simulink model "pre4"  (R2021a)
settings: Solver=VariableStepAuto  StartTime=0.0  StopTime=10.0  RelTol=1e-3
libraries: dsparch4 x3, commsynccomp2 x1, spspowerguiLib x1
settings Model: Creator=Dell  LastModifiedBy=Dell

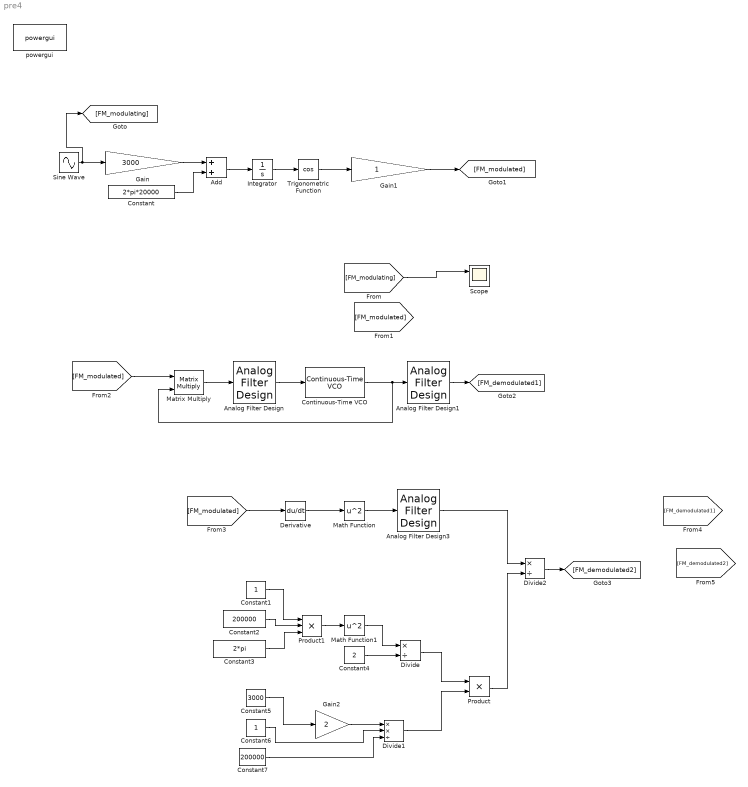
== system pre4 ==
  Add : Sum
  Analog Filter Design : dsparch4/Analog Filter Design  method=Butterworth  filttype=Lowpass  N=8  Wlo=30  Whi=80  Rp=2  Rs=40
  Analog Filter Design1 : dsparch4/Analog Filter Design  method=Butterworth  filttype=Lowpass  N=8  Wlo=30  Whi=80  Rp=2  Rs=40
  Analog Filter Design3 : dsparch4/Analog Filter Design  method=Butterworth  filttype=Bandpass  N=8  Wlo=30  Whi=80  Rp=2  Rs=40
  Constant : Constant  Value=2*pi*20000
  Constant1 : Constant
  Constant2 : Constant  Value=200000
  Constant3 : Constant  Value=2*pi
  Constant4 : Constant  Value=2
  Constant5 : Constant  Value=3000
  Constant6 : Constant
  Constant7 : Constant  Value=200000
  Continuous-Time VCO : commsynccomp2/Continuous-Time VCO  Ac=1  Fc=10  Kc=1  Ph=0
      settings: SourceProductBaseCode=CM
  Derivative : Derivative
  Divide : Product  Inputs=*/
  Divide1 : Product  Inputs=**/
  Divide2 : Product  Inputs=*/
  Gain : Gain  Gain=3000
  Gain1 : Gain
  Gain2 : Gain  Gain=2
  Integrator : Integrator
  Math Function : Math  Operator=square  SaturateOnIntegerOverflow=on
  Math Function1 : Math  Operator=square  SaturateOnIntegerOverflow=on
  Matrix Multiply : Product  Multiplication=Matrix(*)
  Product : Product
  Product1 : Product  Inputs=3
  Scope : Scope  NumInputPorts=2
  Sine Wave : Sin  SampleTime=0
  Trigonometric Function : Trigonometry  Operator=cos
  powergui : spspowerguiLib/powergui  Priority=1  SimulationMode=Continuous  SampleTime=50e-6  frequency=60  Iterations=50  frequencyindice=60  Pbase=100e6  ErrMax=1e-4  UnitsV=kV  UnitsW=MW  buscounter=0  FunctionMessages=off  echomessages=off  EnableUseOfTLC=off  CurrentSourceSwitches=off  DisableSnubberDevices=off  DisableRonSwitches=off  DisableVfSwitches=off  DisplayEquations=off  AutomaticDiscreteSolvers=off  SolverType=Tustin/Backward Euler (TBE)  Interpol=off  ExternalGateDelay=off  methode=off  Ts=100  x0status=blocks  SPID=on  SwTol=0  HookPort=off  NonlinearTolerance=1e-4  nMaxIteration=100  ContinueOnMaxIteration=off  RestoreLinks=warning  ResistiveCurrentMeasurement=off  Frange=[0:2:500]  Ylog=off  Xlog=on  ShowGrid=off  save=off  variable=ZData  structure=0  ZoomFFT=off  StartTime=0.0  cycles=1  DisplayStyle=1  fundamental=60  FreqAxis=off  MaxFrequency=1000  frequencyindicesteady=1  RmsSteady=1  display=off
  wires:
  Sine Wave/1 -> [FM_modulating], Gain/1
  Constant/1 -> Add/2
  Gain/1 -> Add/1
  Add/1 -> Integrator/1
  Integrator/1 -> Trigonometric Function/1
  Trigonometric Function/1 -> Gain1/1
  Gain1/1 -> [FM_modulated]
  [FM_modulating] -> Scope/1
  Analog Filter Design/1 -> Continuous-Time VCO/1
  [FM_modulated] -> Matrix Multiply/1
  Matrix Multiply/1 -> Analog Filter Design/1
  Continuous-Time VCO/1 -> Matrix Multiply/2, Analog Filter Design1/1
  Analog Filter Design1/1 -> [FM_demodulated1]
  [FM_modulated] -> Derivative/1
  Derivative/1 -> Math Function/1
  Math Function/1 -> Analog Filter Design3/1
  Constant1/1 -> Product1/1
  Constant2/1 -> Product1/2
  Constant3/1 -> Product1/3
  Product1/1 -> Math Function1/1
  Math Function1/1 -> Divide/1
  Constant4/1 -> Divide/2
  Divide/1 -> Product/1
  Constant5/1 -> Gain2/1
  Gain2/1 -> Divide1/1
  Constant7/1 -> Divide1/3
  Constant6/1 -> Divide1/2
  Divide1/1 -> Product/2
  Product/1 -> Divide2/2
  Divide2/1 -> [FM_demodulated2]
  Analog Filter Design3/1 -> Divide2/1
